simulink subsystem "full_adder"  (R2019b)
settings: Solver=VariableStepAuto  StartTime=0.0  StopTime=10.0  RelTol=1e-3
settings Model: Creator=prith  LastModifiedBy=prith

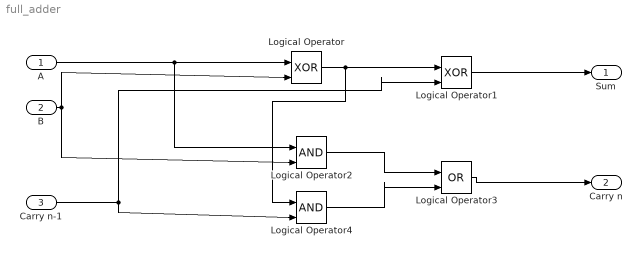
== system full_adder ==
  A : Inport  OutDataTypeStr=boolean
  B : Inport  Port=2  OutDataTypeStr=boolean
  Carry n-1 : Inport  Port=3  OutDataTypeStr=boolean
  Logical Operator : Logic  Operator=XOR  IconShape=distinctive  AllPortsSameDT=off  OutDataTypeStr=boolean
  Logical Operator1 : Logic  Operator=XOR  IconShape=distinctive  AllPortsSameDT=off  OutDataTypeStr=boolean
  Logical Operator2 : Logic  IconShape=distinctive  AllPortsSameDT=off  OutDataTypeStr=boolean
  Logical Operator3 : Logic  Operator=OR  IconShape=distinctive  AllPortsSameDT=off  OutDataTypeStr=boolean
  Logical Operator4 : Logic  IconShape=distinctive  AllPortsSameDT=off  OutDataTypeStr=boolean
  Sum : Outport  OutDataTypeStr=boolean
  Carry n : Outport  Port=2  OutDataTypeStr=boolean
  wires:
  A/1 -> Logical Operator/1, Logical Operator2/1
  B/1 -> Logical Operator2/2, Logical Operator/2
  Carry n-1/1 -> Logical Operator4/2, Logical Operator1/2
  Logical Operator/1 -> Logical Operator1/1, Logical Operator4/1
  Logical Operator2/1 -> Logical Operator3/1
  Logical Operator4/1 -> Logical Operator3/2
  Logical Operator3/1 -> Carry n/1
  Logical Operator1/1 -> Sum/1
